simulink model "Cancelador_de_eco_simplificado"  (R2021b)
settings: Solver=VariableStepAuto  StartTime=0.0  StopTime=10.0  RelTol=1e-3
values from neighbouring files (symbols this model uses):
  T = 1    [Tempo.mat]
settings Model: Creator=duart  LastModifiedBy=duart

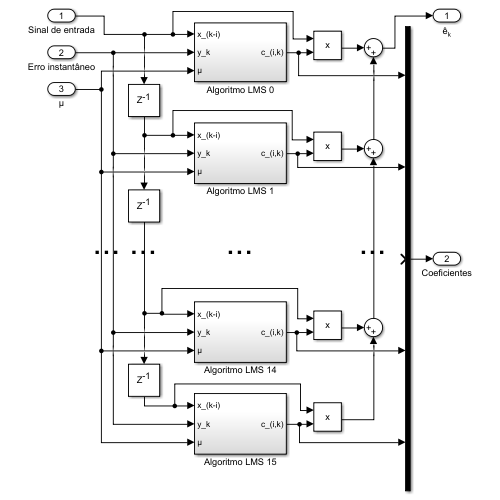
[thumbnail: Simulink's stored preview of the top-level diagram]
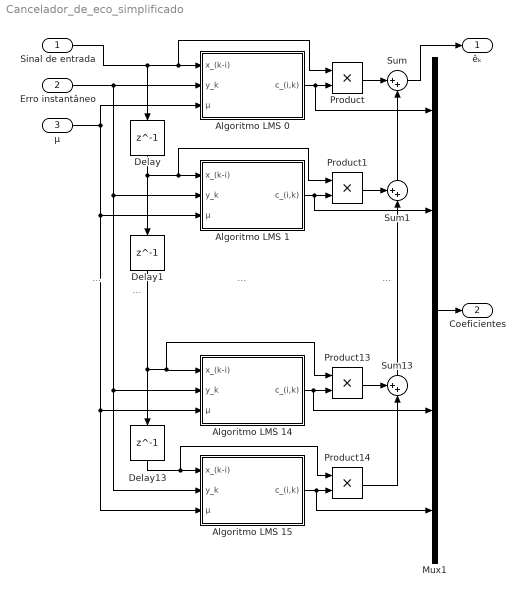
== system Cancelador_de_eco_simplificado ==
  note: ...
  note: ...
  note: ...
  note: ...
  Sinal de entrada : Inport
  Erro instantâneo : Inport  Port=2
  μ : Inport  Port=3
  Algoritmo LMS 0 : Subsystem
  Algoritmo LMS 1 : Subsystem
  Algoritmo LMS 14 : Subsystem
  Algoritmo LMS 15 : Subsystem
  Delay : Delay  DelayLength=1  InitialCondition=0  SampleTime=T
  Delay1 : Delay  DelayLength=1  InitialCondition=0
  Delay13 : Delay  DelayLength=1  InitialCondition=0
  Mux1 : Mux  Inputs=5
  Product{,1,13..14} (4 alike) : Product
  Sum : Sum  Inputs=|++
  Sum1 : Sum  Inputs=++|
  Sum13 : Sum  Inputs=++|
  êₖ : Outport
  Coeficientes : Outport  Port=2
  wires:
  Sinal de entrada/1 -> Product/1, Algoritmo LMS 0/1(x_(k-i)), Delay/1
  Algoritmo LMS 0/1(c_(i,k)) -> Product/2, Mux1/1
  Product/1 -> Sum/1
  Delay/1 -> Product1/1, Algoritmo LMS 1/1(x_(k-i)), Delay1/1
  Algoritmo LMS 1/1(c_(i,k)) -> Mux1/2, Product1/2
  Product1/1 -> Sum1/1
  Product13/1 -> Sum13/1
  Algoritmo LMS 14/1(c_(i,k)) -> Mux1/4, Product13/2
  Delay1/1 -> Product13/1, Algoritmo LMS 14/1(x_(k-i)), Delay13/1
  Product14/1 -> Sum13/2
  Delay13/1 -> Product14/1, Algoritmo LMS 15/1(x_(k-i))
  μ/1 -> Algoritmo LMS 0/3(μ), Algoritmo LMS 14/3(μ), Algoritmo LMS 15/3(μ), Algoritmo LMS 1/3(μ)
  Sum1/1 -> Sum/2
  Sum/1 -> êₖ/1
  Algoritmo LMS 15/1(c_(i,k)) -> Mux1/5, Product14/2
  Mux1/1 -> Coeficientes/1
  Sum13/1 -> Sum1/2
  Erro instantâneo/1 -> Algoritmo LMS 14/2(y_k), Algoritmo LMS 15/2(y_k), Algoritmo LMS 1/2(y_k), Algoritmo LMS 0/2(y_k)

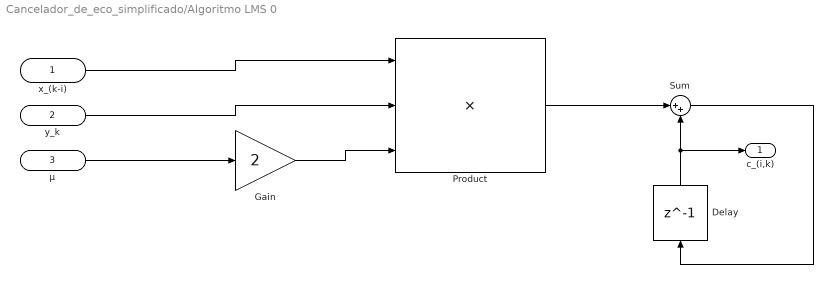
== system Cancelador_de_eco_simplificado/Algoritmo LMS 0 ==
  x_(k-i) : Inport
  y_k : Inport  Port=2
  μ : Inport  Port=3
  Delay : Delay  DelayLength=1  InitialCondition=0  SampleTime=T
  Gain : Gain  Gain=2
  Product : Product  Inputs=3
  Sum : Sum  Inputs=|++
  c_(i,k) : Outport
  wires:
  x_(k-i)/1 -> Product/1
  y_k/1 -> Product/2
  μ/1 -> Gain/1
  Gain/1 -> Product/3
  Product/1 -> Sum/1
  Delay/1 -> c_(i,k)/1, Sum/2
  Sum/1 -> Delay/1

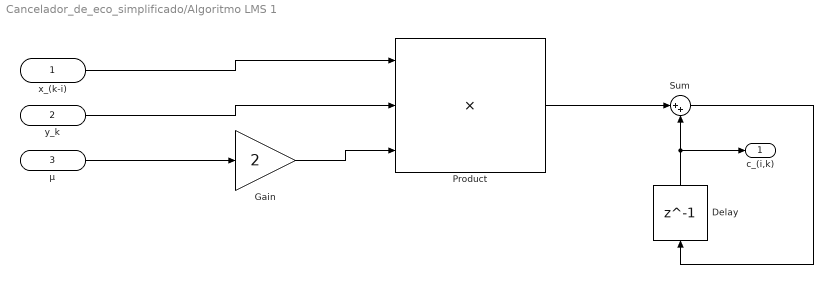
== system Cancelador_de_eco_simplificado/Algoritmo LMS 1 ==
  x_(k-i) : Inport
  y_k : Inport  Port=2
  μ : Inport  Port=3
  Delay : Delay  DelayLength=1  InitialCondition=0  SampleTime=T
  Gain : Gain  Gain=2
  Product : Product  Inputs=3
  Sum : Sum  Inputs=|++
  c_(i,k) : Outport
  wires:
  x_(k-i)/1 -> Product/1
  y_k/1 -> Product/2
  μ/1 -> Gain/1
  Gain/1 -> Product/3
  Product/1 -> Sum/1
  Delay/1 -> c_(i,k)/1, Sum/2
  Sum/1 -> Delay/1

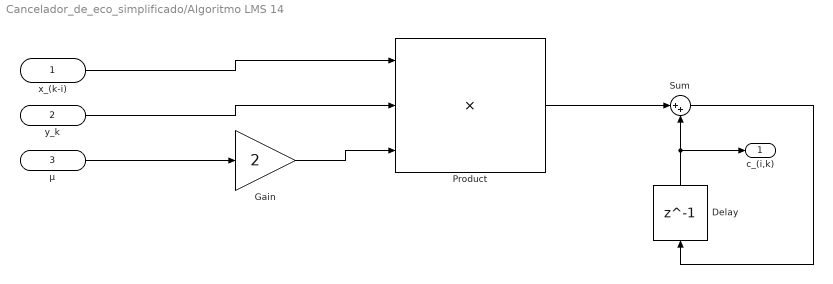
== system Cancelador_de_eco_simplificado/Algoritmo LMS 14 ==
  x_(k-i) : Inport
  y_k : Inport  Port=2
  μ : Inport  Port=3
  Delay : Delay  DelayLength=1  InitialCondition=0  SampleTime=T
  Gain : Gain  Gain=2
  Product : Product  Inputs=3
  Sum : Sum  Inputs=|++
  c_(i,k) : Outport
  wires:
  x_(k-i)/1 -> Product/1
  y_k/1 -> Product/2
  μ/1 -> Gain/1
  Gain/1 -> Product/3
  Product/1 -> Sum/1
  Delay/1 -> c_(i,k)/1, Sum/2
  Sum/1 -> Delay/1

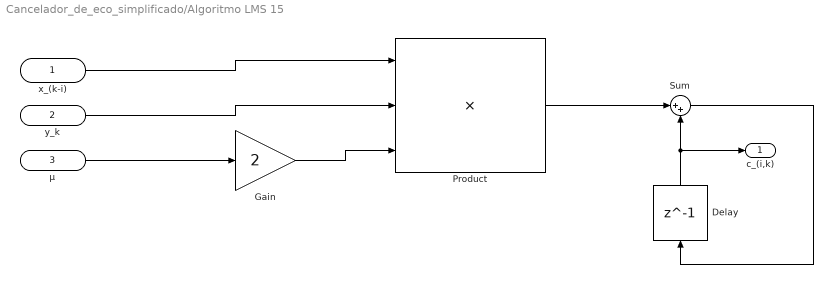
== system Cancelador_de_eco_simplificado/Algoritmo LMS 15 ==
  x_(k-i) : Inport
  y_k : Inport  Port=2
  μ : Inport  Port=3
  Delay : Delay  DelayLength=1  InitialCondition=0  SampleTime=T
  Gain : Gain  Gain=2
  Product : Product  Inputs=3
  Sum : Sum  Inputs=|++
  c_(i,k) : Outport
  wires:
  x_(k-i)/1 -> Product/1
  y_k/1 -> Product/2
  μ/1 -> Gain/1
  Gain/1 -> Product/3
  Product/1 -> Sum/1
  Delay/1 -> c_(i,k)/1, Sum/2
  Sum/1 -> Delay/1
